simulink model "can_simple_block_bu11142"  (R2016b)
settings: Solver=FixedStepDiscrete  StartTime=0.0  StopTime=1000  FixedStep=0.2  RelTol=1e-3  EnableMultiTasking=on
undefined symbols (not defined in the file or in its folder): A, A10, A14, B, B11, B12, B13, B8, C, CS0, D, D11, D4, F3, F4, G3, G4, H3, H4, K17, K4, L3, N16, PA11, PA12, PD0, PE14, PE15, R10, R14, SCK, SIN, SOUT, T14
libraries: rappid_564xl_ec_toolbox x24
(part 1 of 2)
settings Model: Creator=RMuradov  LastModifiedBy=eugkim01
settings SolverCC: AutoInsertRateTranBlk=on
settings DataIOCC: ExternalInput=off  InitialState=off  LimitDataPoints=on  SaveFormat=Array  SignalLoggingSaveFormat=ModelDataLogs  SaveOutput=off  SignalLogging=off  SaveTime=off
settings OptimizationCC: DefaultParameterBehavior=Inlined  UseDivisionForNetSlopeComputation=on  UseFloatMulNetSlope=on  UseSpecifiedMinMax=on  InlineInvariantSignals=on  PassReuseOutputArgsAs=Individual arguments  ExpressionDepthLimit=2147483647  ZeroExternalMemoryAtStartup=off  ZeroInternalMemoryAtStartup=off  NoFixptDivByZeroProtection=on  EfficientFloat2IntCast=on  LifeSpan=1
settings DebuggingCC: UnderspecifiedInitializationDetection=Classic  MergeDetectMultiDrivingBlocksExec=none  SolverPrmCheckMsg=warning  InheritedTsInSrcMsg=none  SingleTaskRateTransMsg=error  ParameterTunabilityLossMsg=error  FcnCallInpInsideContextMsg=warning  UnconnectedInputMsg=error  UnconnectedOutputMsg=error  UnconnectedLineMsg=error  UnknownTsInhSupMsg=error  StateNameClashWarn=warning  SFUnexpectedBacktrackingDiag=warning  SFNoUnconditionalDefaultTransitionDiag=warning  SFExecutionAtInitializationDiag=none
settings HardwareCC: ProdBitPerPointer=32  ProdBitPerSizeT=32  ProdBitPerPtrDiffT=32  ProdLargestAtomicInteger=Long  ProdLargestAtomicFloat=Double  ProdEndianess=BigEndian  ProdWordSize=32  ProdHWDeviceType=Freescale->32-bit PowerPC
settings ModelReferenceCC: PropagateSignalLabelsOutOfModel=off
settings RTWCC: SystemTargetFile=rappid564xl.tlc  MakeCommand=rappid_564xl_make_rtw  TemplateMakefile=rappid_564xl_default_tmf  PostCodeGenCommand=rappid_analyzegencode(buildInfo)  Description=RAppID Toolbox MPC564xL Code Generation Target (rappid)  GenerateReport=on  TLCAssert=on  BuildConfiguration=Faster Runs  IncludeHyperlinkInReport=on  LaunchReport=on  GenerateTraceInfo=on  GenerateTraceReport=on  GenerateTraceReportSl=on  GenerateTraceReportSf=on  GenerateTraceReportEml=on  GenerateCodeMetricsReport=on
settings CodeAppCC: ForceParamTrailComments=on  IgnoreCustomStorageClasses=off  OperatorAnnotations=on  SimulinkDataObjDesc=on  SFDataObjDesc=on  MATLABFcnDesc=on  CustomSymbolStrGlobalVar=rt$N$M  CustomSymbolStrType=$N$M  CustomSymbolStrFcn=$N$M$F  CustomSymbolStrMacro=$N$M  InsertBlockDesc=on  MATLABSourceComments=on  InternalIdentifier=Classic
settings STFCustomTargetCC: CombineOutputUpdateFcns=on  CombineSignalStateStructs=on  ERTCustomFileBanners=on  SupportAbsoluteTime=off  SupportComplex=off  SupportContinuousTime=off  RemoveResetFunc=on  MATLABClassNameForMDSCustomization=Simulink.SoftwareTarget.ERTCustomization  GRTInterface=off  SystemTargetFile=rappid564xl.tlc
settings ERTTargetCC: ParMdlRefBuildCompliant=off  CompOptLevelCompliant=off  ConcurrentExecutionCompliant=off  CombineSignalStateStructs=on  ERTFirstTimeCompliant=off  SupportAbsoluteTime=off  SupportComplex=off  SupportNonInlinedSFcns=on  ModelStepFunctionPrototypeControlCompliant=off  CPPClassGenCompliant=off  UseToolchainInfoCompliant=off  InlinedParameterPlacement=NonHierarchical  ERTCustomFileTemplate=example_file_process.tlc  ERTFilePackagingFormat=CompactWithDataFile
settings ConfigComp: CovMetricSettings=dw  CovHtmlReporting=on  CovSaveCumulativeToWorkspaceVar=on  CovSaveSingleToWorkspaceVar=on  CovExternalEMLEnable=off

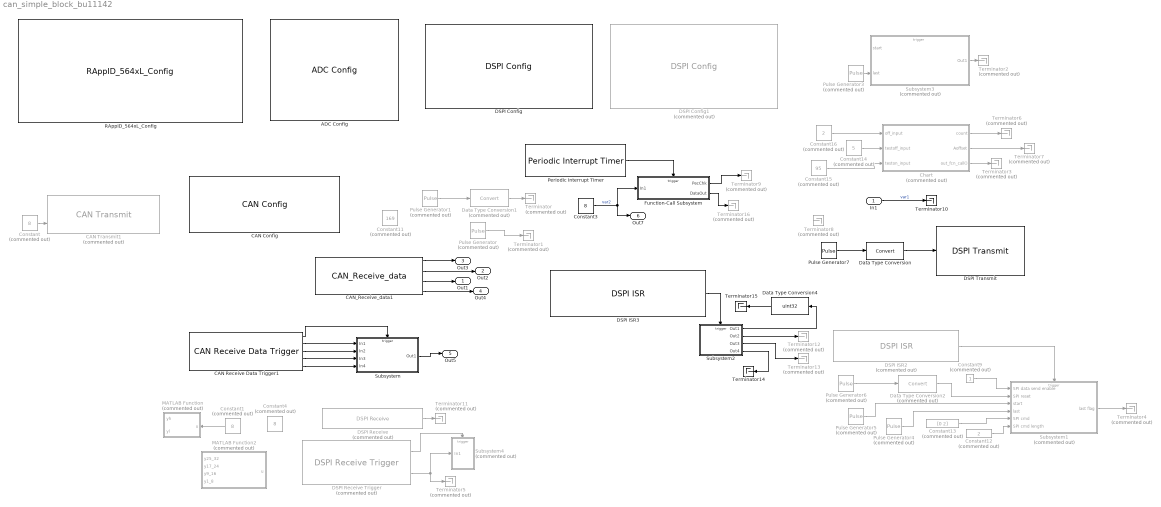
== system can_simple_block_bu11142 ==
  In1 : Inport
  ADC Config : rappid_564xl_ec_toolbox/MPC564xL/Motor Control Blocks/ADC Config  adc_unit=0  adc_ctu=off  adc_owr=on  adc_wls=Left  adc_clk=on  adc_ack=on  adc_ctr0_inp=off  adc_ctr0_shft=10 - Avin = 0  adc_ctr0_cmp=01  adc_ctr0_samp=3  adc_ctr1_inp=off  adc_ctr1_cmp=01  adc_ctr1_samp=1  adc_ctr1_tsens=PTAT  adc_pscr_preval=V0  adc_pscr_preconv=off
  CAN Config : rappid_564xl_ec_toolbox/MPC564xL/Communication Blocks/CAN Config  Priority=1  can_unit=A  can_unit_v2=0  can_idam=A - One full ID (standard or extended) per filter element.  can_srx_dis=1 - Self reception disabled  can_presdiv=4  can_rjw=3  can_pseg1=3  can_pseg2=3  can_clk_src=0 - The CAN engine clock source is the oscillator clock  can_lpb=0 - Loop Back disabled  can_smp=1 - Three samples are used to determine the value of the received bit  can_boff_rec=0 - Automatic recovering from Bus Off state enabled  can_tsyn=0 - Timer Sync feature disabled  can_lbuf=0 - Buffer with highest priority is transmitted first  can_lom=0 - Listen Only Mode is deactivated  can_propseg=6
  CAN Receive Data Trigger1 : rappid_564xl_ec_toolbox/MPC564xL/Communication Blocks/CAN Receive Data Trigger  can_unit=A  can_unit_v2=0  can_buffer=5  can_id=1021  can_isr_prio=14
  CAN Transmit1 : rappid_564xl_ec_toolbox/MPC564xL/Communication Blocks/CAN Transmit  Commented=on  can_unit=A  can_unit_v2=0  can_buffer=14  can_id=522
  CAN_Receive_data1 : rappid_564xl_ec_toolbox/MPC564xL/Communication Blocks/CAN_Receive_data  can_unit=A  can_unit_v2=0  can_buffer=7  can_id=1010
  Chart : Stateflow chart  Commented=on  TreatAsAtomicUnit=on
  Constant : Constant  Commented=on  Value=8  OutDataTypeStr=uint8
  Constant1 : Constant  Commented=on  Value=8  OutDataTypeStr=uint16
  Constant11 : Constant  Commented=on  Value=169  OutDataTypeStr=uint16
  Constant12 : Constant  Commented=on  Value=2  OutDataTypeStr=uint8
  Constant13 : Constant  Commented=on  Value=[0 2]  OutDataTypeStr=uint8
  Constant14 : Constant  Commented=on  Value=5
  Constant15 : Constant  Commented=on  Value=95
  Constant16 : Constant  Commented=on  Value=2
  Constant3 : Constant  Value=8  OutDataTypeStr=uint16
  Constant4 : Constant  Commented=on  Value=8  OutDataTypeStr=uint16
  Constant9 : Constant  Commented=on  OutDataTypeStr=boolean
  DSPI Config : rappid_564xl_ec_toolbox/MPC564xL/Communication Blocks/DSPI Config  Priority=1  dspi_Num=1  dspi_Mode=Master  dspi_MTFE=off  dspi_CONT_SCKE=off  dspi_PCSSE=off  dspi_ROOE=off  dspi_DIS_TXF=Disable  dspi_DIS_RXF_v2=Disable  dspi_SMPL_PT=DSPI samples SIN at driving SCK edge  dspi_FMSZ=8  dspi_CPOL=High  dspi_CPHA=Data is changed on the leading edge of SCK and captured on the following edge  dspi_LSBFE=MSB first  dspi_DBR=off  dspi_PCSSCK=7  dspi_PASC=1  dspi_PDT=5  dspi_PBR=3  dspi_CSSCK=256  dspi_ASC=256  dspi_DT=8  dspi_BR=128  dspi_PCSIS0=High  dspi_PCSIS1=High  dspi_PCSIS2=High  dspi_PCSIS3=High  dspi_PCSIS4=High  dspi_PCSIS5=High  dspi_PCSIS6=High  dspi_PCSIS7=High  dspi_DIS_RXF=Oops
  DSPI Config1 : rappid_564xl_ec_toolbox/MPC564xL/Communication Blocks/DSPI Config  Priority=1  Commented=on  dspi_Num=0  dspi_Mode=Master  dspi_MTFE=off  dspi_CONT_SCKE=off  dspi_PCSSE=off  dspi_ROOE=off  dspi_DIS_TXF=Disable  dspi_DIS_RXF_v2=Disable  dspi_SMPL_PT=DSPI samples SIN at driving SCK edge  dspi_FMSZ=8  dspi_CPOL=Low  dspi_CPHA=Data is changed on the leading edge of SCK and captured on the following edge  dspi_LSBFE=MSB first  dspi_DBR=off  dspi_PCSSCK=1  dspi_PASC=1  dspi_PDT=3  dspi_PBR=1  dspi_CSSCK=8  dspi_ASC=8  dspi_DT=16  dspi_BR=2  dspi_PCSIS0=High  dspi_PCSIS1=High  dspi_PCSIS2=High  dspi_PCSIS3=High  dspi_PCSIS4=High  dspi_PCSIS5=High  dspi_PCSIS6=High  dspi_PCSIS7=High  dspi_DIS_RXF=Oops
  DSPI ISR2 : rappid_564xl_ec_toolbox/MPC564xL/Communication Blocks/DSPI ISR  Commented=on  dspi_Num=1  dspi_isr_name=TCF - Transfer Complete  dspi_isrPrio=13  dspi_isr_tfuf=off  dspi_isr_rfof=on
  DSPI ISR3 : rappid_564xl_ec_toolbox/MPC564xL/Communication Blocks/DSPI ISR  dspi_Num=1  dspi_isr_name=EOQF - End of Queue  dspi_isrPrio=11  dspi_isr_tfuf=off  dspi_isr_rfof=on
  DSPI Receive : rappid_564xl_ec_toolbox/MPC564xL/Communication Blocks/DSPI Receive  Commented=on  dspi_Num=1
  DSPI Receive Trigger : rappid_564xl_ec_toolbox/MPC564xL/Communication Blocks/DSPI Receive Trigger  Commented=on  dspi_Num=1  dspi_ISRPri=13
  DSPI Transmit : rappid_564xl_ec_toolbox/MPC564xL/Communication Blocks/DSPI Transmit  Priority=2  dspi_Num=1  dspi_CONT=off  dspi_PUSHR_PE=off  dspi_PUSHR_PP=off  dspi_PCS_0=36 : C[4] : [11] : [H3] : CS0  dspi_PCS_1=5 : A[5] : [14] : [H4] : CS0  dspi_PCS_2=3 : A[3] : [92] : [K17] : CS0  dspi_PCS_slave_0=36 : C[4] : [11] : [H3] : CS0  dspi_PCS_slave_1=5 : A[5] : [14] : [H4] : CS0  dspi_PCS_slave_2=3 : A[3] : [92] : [K17] : CS0  dspi_SIN_0=39 : C[7] : [15] : [K4] : SIN  dspi_SIN_1=8 : A[8] : [12] : [F4]  dspi_SIN_2=2 : A[2] : [84] : [N16] : SIN  dspi_SCK_0=37 : C[5] : [13] : [G3] : SCK  dspi_SCK_1=6 : A[6] : [2] : [G4] : SCK  dspi_SCK_2=0 : A[0] : [73] : [T14] : SCK  dspi_SOUT_0=38 : C[6] : [142] : [D4] : SOUT  dspi_SOUT_1=7 : A[7] : [10] : [F3] : SOUT  dspi_SOUT_2=1 : A[1] : [74] : [R14] : SOUT  dspi_Strobe=None  dspi_eoq=off  dspi_pcsx=Assert
  Data Type Conversion : DataTypeConversion  Priority=1
  Data Type Conversion1 : DataTypeConversion  Priority=1  Commented=on
  Data Type Conversion2 : DataTypeConversion  Priority=1  Commented=on
  Data Type Conversion4 : DataTypeConversion  Priority=1  OutDataTypeStr=uint32
  Function-Call Subsystem : Subsystem  TreatAsAtomicUnit=on
      settings: RTWSystemCode=Nonreusable function
  MATLAB Function : MATLAB Function  Commented=on  TreatAsAtomicUnit=on
  MATLAB Function2 : MATLAB Function  Commented=on  TreatAsAtomicUnit=on
  Periodic Interrupt Timer : rappid_564xl_ec_toolbox/MPC564xL/General Purpose Blocks/Periodic Interrupt Timer  pit_chan=1  pit_timeout=50  int_priority=12  pit_timeout_val=5999999
  Pulse Generator : DiscretePulseGenerator  Commented=on  Amplitude=9  Period=10
  Pulse Generator1 : DiscretePulseGenerator  Commented=on  Period=5  PulseWidth=3
  Pulse Generator3 : DiscretePulseGenerator  Commented=on  Period=100  PhaseDelay=5
  Pulse Generator4 : DiscretePulseGenerator  Commented=on  Period=100  PhaseDelay=5
  Pulse Generator5 : DiscretePulseGenerator  Commented=on  Period=100
  Pulse Generator6 : DiscretePulseGenerator  Commented=on  Period=10000000  PhaseDelay=1
  Pulse Generator7 : DiscretePulseGenerator  Amplitude=0  Period=100
  RAppID_564xL_Config : rappid_564xl_ec_toolbox/MPC564xL/RAppID_564xL_Config  SystemClock=120  XTAL=40  MC_clock_60=12  MC_clock_80=16  MC_clock_120=10  SWG_clock_60=20  SWG_clock_80=13.334  SWG_clock_120=20  Compiler=CodeWarrior  MemTarget=RAM  Part=MPC5643L  Package=144 LQFP  global_int_priority=11  base_tick_priority=12  sys_task_supress=off  exception_handlers=off  stored_mdl_name=can_simple_block_bu11142  freemaster_interface=Oops  freemaster_rx_pin="LINFlex_0 Rx Pin 116 : \"PB[3]\""  freemaster_tx_pin="LINFlex_0 Tx Pin 114 : \"PB[2]\""  freemaster_interface_1=None  freemaster_enable=off  freemaster_rate=57600  freemaster_tx0_pin=18 : B[2] : 114 : A14  freemaster_rx0_pin=19 : B[3] : 116 : B13  freemaster_tx1_pin=57 : D[9] : 26 : L3  freemaster_rx1_pin=29 : B[13] : 60 : R10  freemaster_can_channel=1CH  freemater_can_speed=500K  freemaster_can_msgig=0x7AA  ccp_interface=None  ccp_enable=off  ccp_can_channel=CH1 (MB 0 - 1)  ccp_can_speed=500K  ccp_can_cro_id=256  ccp_can_dto_id=257  ccp_dev_id=RappID  ccp_dev_addr=0  ccp_odt=3  ccp_daq=3  pil_enable=off  pil_bam=on  comport=6  pil_rate=57600  bam_password_def=on  bam_password=0xFEEDFACECAFEBEEF  bam_sa_cs=on  bam_start_address=0x40005000  bam_code_size=0xa000  cons_dspi=on  cons_can=on  cons_adc=on  cons_pwm=on  cons_ctu=on  cons_swg=on  cons_eTimer=on  cons_fm=on
  Subsystem : Subsystem
      settings: RTWSystemCode=Nonreusable function
  Subsystem1 : Subsystem  Commented=on
      settings: RTWSystemCode=Nonreusable function
  Subsystem2 : Subsystem
      settings: RTWSystemCode=Nonreusable function
  Subsystem3 : Subsystem  Commented=on
  Subsystem4 : Subsystem  Commented=on
      settings: RTWSystemCode=Nonreusable function
  Terminator{,1..9,11..13,16} (14 alike) : Terminator  Commented=on
  Terminator10 : Terminator
  Terminator14 : Terminator
  Terminator15 : Terminator
  Out1 : Outport
  Out2 : Outport  Port=2
  Out3 : Outport  Port=3
  Out4 : Outport  Port=4
  Out5 : Outport  Port=5
  Out7 : Outport  Port=6
  wires:
  CAN_Receive_data1/4 -> Out4/1
  CAN_Receive_data1/3 -> Out1/1
  CAN_Receive_data1/2 -> Out2/1
  CAN_Receive_data1/1 -> Out3/1
  Constant/1 -> CAN Transmit1/2
  CAN Receive Data Trigger1/3 -> Subsystem/2(In2)
  CAN Receive Data Trigger1/4 -> Subsystem/3(In3)
  CAN Receive Data Trigger1/5 -> Subsystem/4(In4)
  CAN Receive Data Trigger1/2 -> Subsystem/1(In1)
  CAN Receive Data Trigger1/1 -> Subsystem/Trigger
  Subsystem/1(Out1) -> Out5/1
  Pulse Generator1/1 -> Data Type Conversion1/1
  Data Type Conversion1/1 -> Terminator/1
  DSPI ISR2/1 -> Subsystem1/Trigger
  DSPI ISR3/1 -> Subsystem2/Trigger
  Constant9/1 -> Subsystem1/1(SPI data send enable)
  Pulse Generator/1 -> Terminator1/1
  Subsystem1/1(last flag) -> Terminator4/1
  Pulse Generator3/1 -> Subsystem3/2(last)
  Subsystem3/1(Out1) -> Terminator2/1
  Pulse Generator4/1 -> Subsystem1/4(last)
  Constant12/1 -> Subsystem1/6(SPI cmd length)
  Constant13/1 -> Subsystem1/5(SPI cmd)
  Chart/1(count) -> Terminator6/1
  Chart/2(" Aoffset") -> Terminator7/1
  Constant16/1 -> Chart/1(off_input)
  Constant14/1 -> Chart/2(testoff_input)
  Constant15/1 -> Chart/3(teston_input)
  Pulse Generator5/1 -> Subsystem1/3(start)
  Pulse Generator6/1 -> Data Type Conversion2/1
  Data Type Conversion2/1 -> Subsystem1/2(SPI reset)
  Chart/3(out_fcn_call()) -> Terminator3/1
  Periodic Interrupt Timer/1 -> Function-Call Subsystem/Trigger
  In1/1 -> Terminator10/1  "var1"
  Constant3/1 -> Function-Call Subsystem/1(In1), Out7/1  "var2"
  Data Type Conversion/1 -> DSPI Transmit/1
  Pulse Generator7/1 -> Data Type Conversion/1
  Data Type Conversion4/1 -> Terminator15/1
  DSPI Receive Trigger/2 -> Terminator5/1, Subsystem4/1(In1)
  DSPI Receive Trigger/1 -> Subsystem4/Trigger
  Subsystem2/1(Out1) -> Data Type Conversion4/1
  DSPI Receive/1 -> Terminator11/1
  Subsystem2/4(Out4) -> Terminator14/1
  Subsystem2/2(Out2) -> Terminator12/1
  Subsystem2/3(Out3) -> Terminator13/1
  Constant1/1 -> MATLAB Function/1(u)
  Function-Call Subsystem/1(PecChk) -> Terminator9/1
  Function-Call Subsystem/2(DataOut) -> Terminator16/1

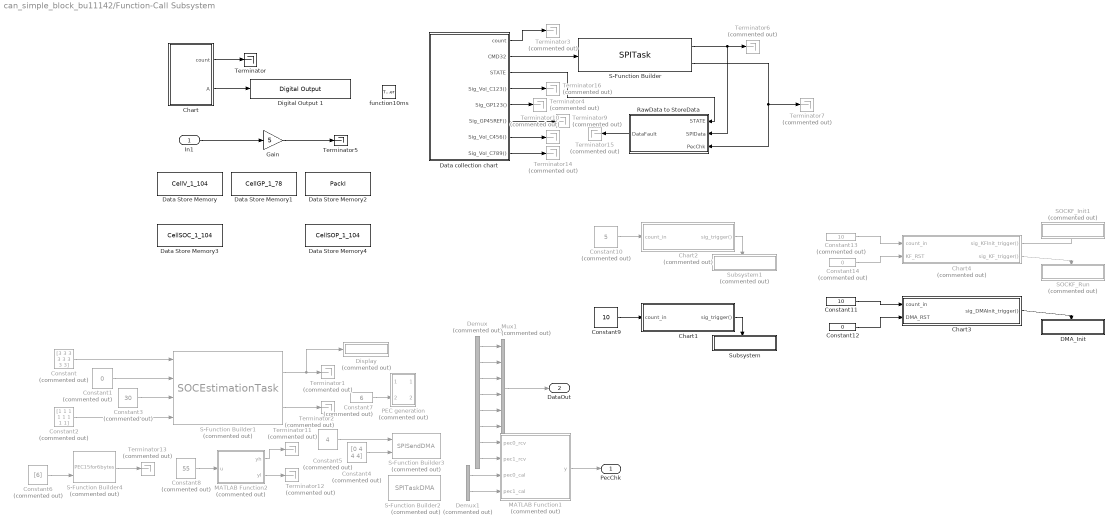
== system can_simple_block_bu11142/Function-Call Subsystem ==
  In1 : Inport
  function10ms : TriggerPort  TriggerType=function-call  VariantControl=Variant
  Chart : Stateflow chart  TreatAsAtomicUnit=on
  Chart1 : Stateflow chart  TreatAsAtomicUnit=on
  Chart2 : Stateflow chart  Commented=on  TreatAsAtomicUnit=on
  Chart3 : Stateflow chart  TreatAsAtomicUnit=on
  Chart4 : Stateflow chart  Commented=on  TreatAsAtomicUnit=on
  Constant : Constant  Commented=on  Value=[3 3 3 3 3 3 3 3]
  Constant1 : Constant  Commented=on  Value=0
  Constant10 : Constant  Commented=on  Value=5  OutDataTypeStr=Inherit: Inherit via back propagation
  Constant11 : Constant  Value=10  OutDataTypeStr=Inherit: Inherit via back propagation
  Constant12 : Constant  Value=0  OutDataTypeStr=Inherit: Inherit via back propagation
  Constant13 : Constant  Commented=on  Value=10  OutDataTypeStr=Inherit: Inherit via back propagation
  Constant14 : Constant  Commented=on  Value=0  OutDataTypeStr=Inherit: Inherit via back propagation
  Constant2 : Constant  Commented=on  Value=[1 1 1 1 1 1 1 1]  OutDataTypeStr=boolean
  Constant3 : Constant  Commented=on  Value=30
  Constant4 : Constant  Commented=on  Value=[0 4 4 4]  OutDataTypeStr=Inherit: Inherit via back propagation
  Constant5 : Constant  Commented=on  Value=4  OutDataTypeStr=Inherit: Inherit via back propagation
  Constant6 : Constant  Commented=on  Value=[6]  OutDataTypeStr=Inherit: Inherit via back propagation
  Constant7 : Constant  Commented=on  Value=6  OutDataTypeStr=Inherit: Inherit via back propagation
  Constant8 : Constant  Commented=on  Value=55  OutDataTypeStr=Inherit: Inherit via back propagation
  Constant9 : Constant  Value=10  OutDataTypeStr=Inherit: Inherit via back propagation
  DMA_Init : Subsystem
  Data Store Memory : DataStoreMemory  DataStoreName=CellV_1_104  ReadBeforeWriteMsg=warning  WriteAfterWriteMsg=warning  WriteAfterReadMsg=warning  ShowAdditionalParam=off  OutDataTypeStr=uint16  Dimensions=104
  Data Store Memory1 : DataStoreMemory  DataStoreName=CellGP_1_78  ReadBeforeWriteMsg=warning  WriteAfterWriteMsg=warning  WriteAfterReadMsg=warning  ShowAdditionalParam=off  OutDataTypeStr=int16  Dimensions=78
  Data Store Memory2 : DataStoreMemory  DataStoreName=PackI  ReadBeforeWriteMsg=warning  WriteAfterWriteMsg=warning  WriteAfterReadMsg=warning  ShowAdditionalParam=off  OutDataTypeStr=int32  Dimensions=1
  Data Store Memory3 : DataStoreMemory  DataStoreName=CellSOC_1_104  ReadBeforeWriteMsg=warning  WriteAfterWriteMsg=warning  WriteAfterReadMsg=warning  ShowAdditionalParam=off  OutDataTypeStr=uint16  Dimensions=104
  Data Store Memory4 : DataStoreMemory  DataStoreName=CellSOP_1_104  ReadBeforeWriteMsg=warning  WriteAfterWriteMsg=warning  WriteAfterReadMsg=warning  ShowAdditionalParam=off  OutDataTypeStr=int16  Dimensions=104
  Data collection chart : Stateflow chart  TreatAsAtomicUnit=on
  Demux : Demux  Commented=on  Outputs=8
  Demux1 : Demux  Commented=on  Outputs=2
  Digital Output 1 : rappid_564xl_ec_toolbox/MPC564xL/General Purpose Blocks/Digital Output   gpio_outputs="78  : PE14 : [ 119 ] : [ B12 ]"  pinNum=[ 119 ]  pcrNum=78
  Display : Display  Commented=on
  Gain : Gain  Gain=5
  MATLAB Function1 : MATLAB Function  Commented=on  TreatAsAtomicUnit=on
  MATLAB Function2 : MATLAB Function  Commented=on  TreatAsAtomicUnit=on
  Mux1 : Mux  Commented=on  Inputs=6
  PEC generation : MATLAB Function  Commented=on  TreatAsAtomicUnit=on
  RawData to StoreData : MATLAB Function  TreatAsAtomicUnit=on
  S-Function Builder : S-Function  InitFcn=try, set_param(gcb,'FunctionName','SPITask'), end  FunctionName=SPITask  SFunctionModules=SPITask_wrapper BMU_Driver  SFunctionDeploymentMode=off  EnableBusSupport=off  mask(S-Function Builder){}
      mask help: Simulink:masks:SFunctionBuilder_MD
      mask init:
      | val = [[.9  0.75 0.75 1 1 .9 .9 1]',[1 1 0.75 0.75 .9 .9 1 .9]'];try , sys = get_param(gcb,'SfunBuilderFcnName');if isempty(sys), sys = get_param(gcb,'FunctionName'); end,catch, sys = get_param(gcb,'FunctionName'); end
      settings: CopyFcn=set_param(gcbh,'LinkStatus','none')  PreSaveFcn=try, set_param(gcb,'FunctionName','SPITask'), end  OpenFcn=sfunctionwizard(gcbh)
      mask Display: plot(val(:,1),val(:,2)),disp(sys), port_label('input',1,'CMD32'), port_label('output',1,'y0'), port_label('output',2,'PecChk')
  S-Function Builder1 : S-Function  Commented=on  InitFcn=try, set_param(gcb,'FunctionName','SOCEstimationTask'), end  FunctionName=SOCEstimationTask  SFunctionModules=SOCEstimationTask_wrapper Extended look2_binlx rtGetNaN rtGetInf rt_nonfinite const_params  SFunctionDeploymentMode=off  EnableBusSupport=off  mask(S-Function Builder){}
      mask help: Simulink:masks:SFunctionBuilder_MD
      mask init: same as can_simple_block_bu11142/Function-Call Subsystem/S-Function Builder
      settings: CopyFcn=set_param(gcbh,'LinkStatus','none')  PreSaveFcn=try, set_param(gcb,'FunctionName','SOCEstimationTask'), end  OpenFcn=sfunctionwizard(gcbh)
      mask Display: plot(val(:,1),val(:,2)),disp(sys), port_label('input',1,'I'), port_label('input',2,'V8'), port_label('input',3,'T'), port_label('input',4,'Enable8'), port_label('output',1,'SOC'), port_label('output',2,'Vt')
  S-Function Builder2 : S-Function  Commented=on  InitFcn=try, set_param(gcb,'FunctionName','SPITaskDMA'), end  FunctionName=SPITaskDMA  SFunctionModules=SPITaskDMA_wrapper BMU_Driver  SFunctionDeploymentMode=off  EnableBusSupport=off  mask(S-Function Builder){}
      mask help: Simulink:masks:SFunctionBuilder_MD
      mask init: same as can_simple_block_bu11142/Function-Call Subsystem/S-Function Builder
      settings: CopyFcn=set_param(gcbh,'LinkStatus','none')  PreSaveFcn=try, set_param(gcb,'FunctionName','SPITaskDMA'), end  OpenFcn=sfunctionwizard(gcbh)
      mask Display: plot(val(:,1),val(:,2)),disp(sys), port_label('output',1,'y0')
  S-Function Builder3 : S-Function  Commented=on  InitFcn=try, set_param(gcb,'FunctionName','SPISendDMA'), end  FunctionName=SPISendDMA  SFunctionModules=SPISendDMA_wrapper DMA  SFunctionDeploymentMode=off  EnableBusSupport=off  mask(S-Function Builder){}
      mask help: Simulink:masks:SFunctionBuilder_MD
      mask init: same as can_simple_block_bu11142/Function-Call Subsystem/S-Function Builder
      settings: CopyFcn=set_param(gcbh,'LinkStatus','none')  PreSaveFcn=try, set_param(gcb,'FunctionName','SPISendDMA'), end  OpenFcn=sfunctionwizard(gcbh)
      mask Display: plot(val(:,1),val(:,2)),disp(sys), port_label('input',1,'len'), port_label('input',2,'data')
  S-Function Builder4 : S-Function  Commented=on  InitFcn=try, set_param(gcb,'FunctionName','PEC15for6bytes'), end  FunctionName=PEC15for6bytes  SFunctionModules=PEC15for6bytes_wrapper BMU_Driver  SFunctionDeploymentMode=off  EnableBusSupport=off  mask(S-Function Builder){}
      mask help: Simulink:masks:SFunctionBuilder_MD
      mask init: same as can_simple_block_bu11142/Function-Call Subsystem/S-Function Builder
      settings: CopyFcn=set_param(gcbh,'LinkStatus','none')  PreSaveFcn=try, set_param(gcb,'FunctionName','PEC15for6bytes'), end  OpenFcn=sfunctionwizard(gcbh)
      mask Display: plot(val(:,1),val(:,2)),disp(sys), port_label('input',1,'data'), port_label('input',2,'len'), port_label('output',1,'y0')
  SOCKF_Init1 : Subsystem  Commented=on
  SOCKF_Run : Subsystem  Commented=on
  Subsystem : Subsystem
  Subsystem1 : Subsystem  Commented=on
  Terminator : Terminator
  Terminator{1..4,6..7,9..16} (14 alike) : Terminator  Commented=on
  Terminator5 : Terminator
  PecChk : Outport
  DataOut : Outport  Port=2
  wires:
  In1/1 -> Gain/1
  Gain/1 -> Terminator5/1
  Chart/2(" A") -> Digital Output 1/1
  Chart/1(count) -> Terminator/1
  S-Function Builder/1 -> RawData to StoreData/2(SPIData), Terminator6/1
  S-Function Builder1/1 -> Terminator1/1, Display/1
  S-Function Builder1/2 -> Terminator2/1
  Constant/1 -> S-Function Builder1/1
  Constant1/1 -> S-Function Builder1/2
  Constant2/1 -> S-Function Builder1/4
  Constant3/1 -> S-Function Builder1/3
  Constant4/1 -> S-Function Builder3/2
  Constant5/1 -> S-Function Builder3/1
  Constant6/1 -> S-Function Builder4/2
  Demux/7 -> MATLAB Function1/1(pec0_rcv)
  Demux/8 -> MATLAB Function1/2(pec1_rcv)
  MATLAB Function1/1(y) -> PecChk/1
  Demux/1 -> Mux1/1
  Demux/2 -> Mux1/2
  Demux/3 -> Mux1/3
  Demux/4 -> Mux1/4
  Demux/5 -> Mux1/5
  Demux/6 -> Mux1/6
  S-Function Builder4/1 -> Terminator13/1
  Mux1/1 -> DataOut/1
  Constant7/1 -> PEC generation/2(len)
  MATLAB Function2/1(yh) -> Terminator11/1
  MATLAB Function2/2(yl) -> Terminator12/1
  Constant8/1 -> MATLAB Function2/1(u)
  S-Function Builder/2 -> Terminator7/1, RawData to StoreData/3(PecChk)
  Demux1/1 -> MATLAB Function1/3(pec0_cal)
  Demux1/2 -> MATLAB Function1/4(pec1_cal)
  Data collection chart/1(count) -> Terminator3/1
  Data collection chart/2(CMD32) -> S-Function Builder/1
  Data collection chart/3(STATE) -> RawData to StoreData/1(STATE)
  Data collection chart/5(Sig_GP123()) -> Terminator4/1
  Data collection chart/6(Sig_GP45REF()) -> Terminator9/1
  Data collection chart/7(Sig_Vol_C456()) -> Terminator10/1
  Data collection chart/8(Sig_Vol_C789()) -> Terminator14/1
  RawData to StoreData/1(DataFault) -> Terminator15/1
  Data collection chart/4(Sig_Vol_C123()) -> Terminator16/1
  Constant9/1 -> Chart1/1(count_in)
  Chart1/1(sig_trigger()) -> Subsystem/Trigger
  Constant10/1 -> Chart2/1(count_in)
  Chart2/1(sig_trigger()) -> Subsystem1/Trigger
  Chart3/1(sig_DMAInit_trigger()) -> DMA_Init/Trigger
  Constant11/1 -> Chart3/1(count_in)
  Constant12/1 -> Chart3/2(DMA_RST)
  Chart4/1(sig_KFInit_trigger()) -> SOCKF_Init1/Trigger
  Constant13/1 -> Chart4/1(count_in)
  Constant14/1 -> Chart4/2(KF_RST)
  Chart4/2(sig_KF_trigger()) -> SOCKF_Run/Trigger

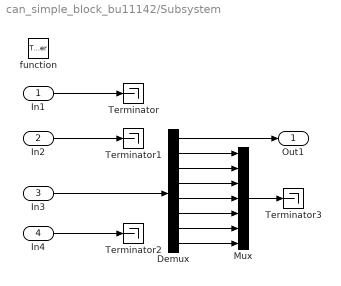
== system can_simple_block_bu11142/Subsystem ==
  In1 : Inport
  In2 : Inport  Port=2
  In3 : Inport  Port=3
  In4 : Inport  Port=4
  function : TriggerPort  TriggerType=function-call  VariantControl=Variant
  Demux : Demux  Outputs=8
  Mux : Mux  Inputs=7
  Terminator{,1..3} (4 alike) : Terminator
  Out1 : Outport
  wires:
  In1/1 -> Terminator/1
  In2/1 -> Terminator1/1
  In4/1 -> Terminator2/1
  In3/1 -> Demux/1
  Demux/8 -> Mux/7
  Demux/7 -> Mux/6
  Demux/6 -> Mux/5
  Demux/5 -> Mux/4
  Demux/4 -> Mux/3
  Demux/3 -> Mux/2
  Demux/2 -> Mux/1
  Mux/1 -> Terminator3/1
  Demux/1 -> Out1/1

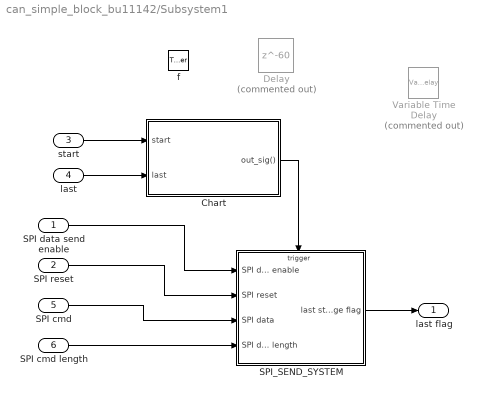
== system can_simple_block_bu11142/Subsystem1 ==
  SPI data send enable : Inport
  SPI reset : Inport  Port=2
  start : Inport  Port=3
  last : Inport  Port=4
  SPI cmd : Inport  Port=5
  SPI cmd length : Inport  Port=6
  f : TriggerPort  TriggerType=function-call  VariantControl=Variant
  Chart : Stateflow chart  TreatAsAtomicUnit=on
  Delay : Delay  Commented=on  DelayLength=60  InitialCondition=0
  SPI_SEND_SYSTEM : Subsystem
  Variable Time Delay : VariableTransportDelay  Commented=on  MaximumDelay=10
  last flag : Outport
  wires:
  SPI data send enable/1 -> SPI_SEND_SYSTEM/1(SPI data send enable)
  SPI reset/1 -> SPI_SEND_SYSTEM/2(SPI reset)
  SPI_SEND_SYSTEM/1(last stage flag) -> last flag/1
  start/1 -> Chart/1(start)
  last/1 -> Chart/2(last)
  SPI cmd/1 -> SPI_SEND_SYSTEM/3(SPI data)
  SPI cmd length/1 -> SPI_SEND_SYSTEM/4(SPI data length)
  Chart/1(out_sig()) -> SPI_SEND_SYSTEM/Trigger

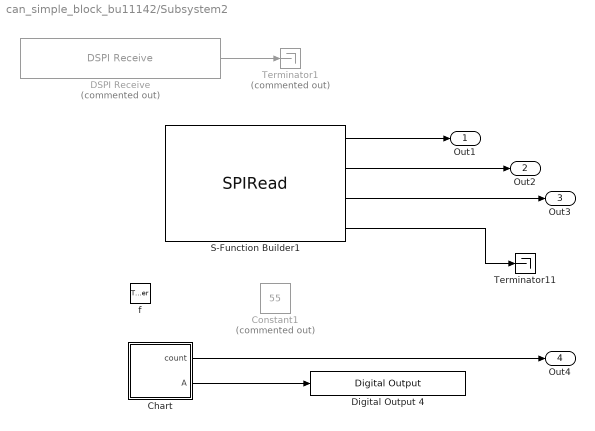
== system can_simple_block_bu11142/Subsystem2 ==
  f : TriggerPort  TriggerType=function-call  VariantControl=Variant
  Chart : Stateflow chart  TreatAsAtomicUnit=on
  Constant1 : Constant  Commented=on  Value=55  OutDataTypeStr=uint16
  DSPI Receive : rappid_564xl_ec_toolbox/MPC564xL/Communication Blocks/DSPI Receive  Commented=on  dspi_Num=1
  Digital Output 4 : rappid_564xl_ec_toolbox/MPC564xL/General Purpose Blocks/Digital Output   gpio_outputs="12  : PA12 : [ 122 ] : [ A10 ]"  pinNum=[ 122 ]  pcrNum=12
  S-Function Builder1 : S-Function  InitFcn=try, set_param(gcb,'FunctionName','SPIRead'), end  FunctionName=SPIRead  SFunctionModules=SPIRead_wrapper BMU_Driver  SFunctionDeploymentMode=off  EnableBusSupport=off  mask(S-Function Builder){}
      mask help: Simulink:masks:SFunctionBuilder_MD
      mask init: same as can_simple_block_bu11142/Function-Call Subsystem/S-Function Builder
      settings: CopyFcn=set_param(gcbh,'LinkStatus','none')  PreSaveFcn=try, set_param(gcb,'FunctionName','SPIRead'), end  OpenFcn=sfunctionwizard(gcbh)
      mask Display: plot(val(:,1),val(:,2)),disp(sys), port_label('output',1,'Vc1'), port_label('output',2,'Vc2'), port_label('output',3,'Vc3'), port_label('output',4,'PEC')
  Terminator1 : Terminator  Commented=on
  Terminator11 : Terminator
  Out1 : Outport
  Out2 : Outport  Port=2
  Out3 : Outport  Port=3
  Out4 : Outport  Port=4
  wires:
  Chart/2(" A") -> Digital Output 4/1
  Chart/1(count) -> Out4/1
  DSPI Receive/1 -> Terminator1/1
  S-Function Builder1/1 -> Out1/1
  S-Function Builder1/2 -> Out2/1
  S-Function Builder1/3 -> Out3/1
  S-Function Builder1/4 -> Terminator11/1

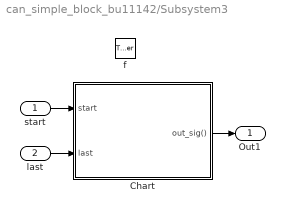
== system can_simple_block_bu11142/Subsystem3 ==
  start : Inport
  last : Inport  Port=2
  f : TriggerPort  TriggerType=function-call  VariantControl=Variant
  Chart : Stateflow chart  TreatAsAtomicUnit=on
  Out1 : Outport
  wires:
  start/1 -> Chart/1(start)
  last/1 -> Chart/2(last)
  Chart/1(out_sig()) -> Out1/1

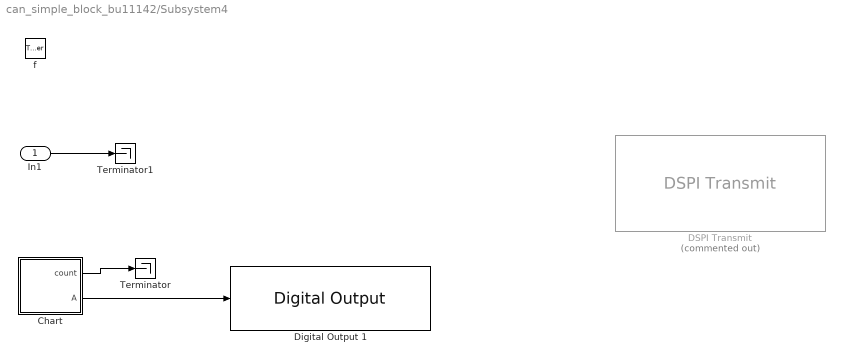
== system can_simple_block_bu11142/Subsystem4 ==
  In1 : Inport
  f : TriggerPort  TriggerType=function-call  VariantControl=Variant
  Chart : Stateflow chart  TreatAsAtomicUnit=on
  DSPI Transmit : rappid_564xl_ec_toolbox/MPC564xL/Communication Blocks/DSPI Transmit  Priority=2  Commented=on  dspi_Num=0  dspi_CONT=off  dspi_PUSHR_PE=off  dspi_PUSHR_PP=off  dspi_PCS_0=36 : C[4] : [11] : [H3] : CS0  dspi_PCS_1=5 : A[5] : [14] : [H4] : CS0  dspi_PCS_2=3 : A[3] : [92] : [K17] : CS0  dspi_PCS_slave_0=36 : C[4] : [11] : [H3] : CS0  dspi_PCS_slave_1=5 : A[5] : [14] : [H4] : CS0  dspi_PCS_slave_2=3 : A[3] : [92] : [K17] : CS0  dspi_SIN_0=39 : C[7] : [15] : [K4] : SIN  dspi_SIN_1=8 : A[8] : [12] : [F4]  dspi_SIN_2=2 : A[2] : [84] : [N16] : SIN  dspi_SCK_0=37 : C[5] : [13] : [G3] : SCK  dspi_SCK_1=6 : A[6] : [2] : [G4] : SCK  dspi_SCK_2=0 : A[0] : [73] : [T14] : SCK  dspi_SOUT_0=38 : C[6] : [142] : [D4] : SOUT  dspi_SOUT_1=7 : A[7] : [10] : [F3] : SOUT  dspi_SOUT_2=1 : A[1] : [74] : [R14] : SOUT  dspi_Strobe=None  dspi_eoq=off  dspi_pcsx=Assert
  Digital Output 1 : rappid_564xl_ec_toolbox/MPC564xL/General Purpose Blocks/Digital Output   gpio_outputs="79  : PE15 : [ 121 ] : [ B11 ]"  pinNum=[ 121 ]  pcrNum=79
  Terminator : Terminator
  Terminator1 : Terminator
  wires:
  In1/1 -> Terminator1/1
  Chart/1(count) -> Terminator/1
  Chart/2(" A") -> Digital Output 1/1

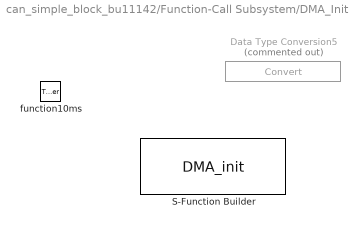
== system can_simple_block_bu11142/Function-Call Subsystem/DMA_Init ==
  function10ms : TriggerPort  TriggerType=function-call  VariantControl=Variant
  Data Type Conversion5 : DataTypeConversion  Priority=1  Commented=on
  S-Function Builder : S-Function  InitFcn=try, set_param(gcb,'FunctionName','DMA_init'), end  FunctionName=DMA_init  SFunctionModules=DMA_init_wrapper DMA  SFunctionDeploymentMode=off  EnableBusSupport=off  mask(S-Function Builder){}
      mask help: Simulink:masks:SFunctionBuilder_MD
      mask init: same as can_simple_block_bu11142/Function-Call Subsystem/S-Function Builder
      settings: CopyFcn=set_param(gcbh,'LinkStatus','none')  PreSaveFcn=try, set_param(gcb,'FunctionName','DMA_init'), end  OpenFcn=sfunctionwizard(gcbh)
      mask Display:
      | plot(val(:,1),val(:,2))
      | disp(sys)

== system can_simple_block_bu11142/Function-Call Subsystem/SOCKF_Init1 ==
  function10ms : TriggerPort  TriggerType=function-call  VariantControl=Variant
  Data Type Conversion5 : DataTypeConversion  Priority=1  Commented=on
  S-Function Builder1 : S-Function  InitFcn=try, set_param(gcb,'FunctionName','SOCEstimationInit'), end  FunctionName=SOCEstimationInit  SFunctionModules=SOCEstimationInit_wrapper Extended look2_binlx rtGetNaN rtGetInf rt_nonfinite const_params rt_roundd_snf  SFunctionDeploymentMode=off  EnableBusSupport=off  mask(S-Function Builder){}
      mask help: Simulink:masks:SFunctionBuilder_MD
      mask init: same as can_simple_block_bu11142/Function-Call Subsystem/S-Function Builder
      settings: CopyFcn=set_param(gcbh,'LinkStatus','none')  PreSaveFcn=try, set_param(gcb,'FunctionName','SOCEstimationInit'), end  OpenFcn=sfunctionwizard(gcbh)
      mask Display:
      | plot(val(:,1),val(:,2))
      | disp(sys)

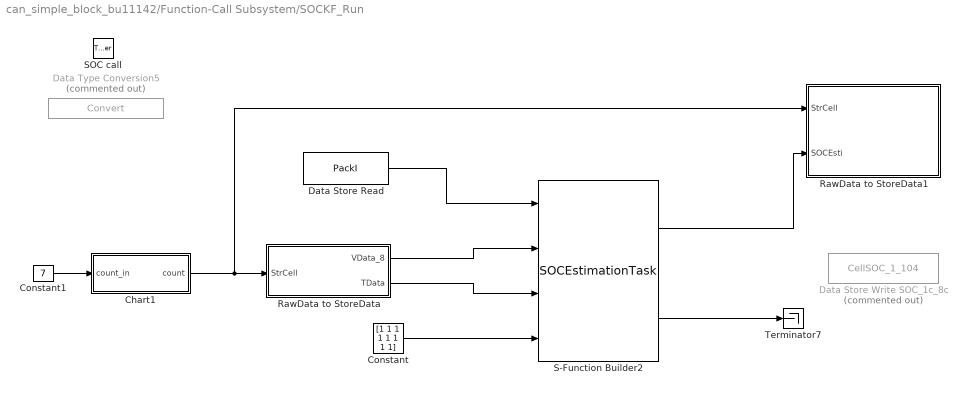
== system can_simple_block_bu11142/Function-Call Subsystem/SOCKF_Run ==
  SOC call : TriggerPort  TriggerType=function-call  VariantControl=Variant
  Chart1 : Stateflow chart  TreatAsAtomicUnit=on
  Constant : Constant  Value=[1 1 1 1 1 1 1 1]  OutDataTypeStr=Inherit: Inherit via back propagation
  Constant1 : Constant  Value=7  OutDataTypeStr=uint8
  Data Store Read : DataStoreRead  DataStoreName=PackI
  Data Store Write SOC_1c_8c : DataStoreWrite  Commented=on  DataStoreName=CellSOC_1_104
  Data Type Conversion5 : DataTypeConversion  Priority=1  Commented=on
  RawData to StoreData : MATLAB Function  TreatAsAtomicUnit=on
  RawData to StoreData1 : MATLAB Function  TreatAsAtomicUnit=on
  S-Function Builder2 : S-Function  InitFcn=try, set_param(gcb,'FunctionName','SOCEstimationTask'), end  FunctionName=SOCEstimationTask  SFunctionModules=SOCEstimationTask_wrapper Extended look2_binlx rtGetNaN rtGetInf rt_nonfinite const_params rt_roundd_snf  SFunctionDeploymentMode=off  EnableBusSupport=off  mask(S-Function Builder){}
      mask help: Simulink:masks:SFunctionBuilder_MD
      mask init: same as can_simple_block_bu11142/Function-Call Subsystem/S-Function Builder
      settings: CopyFcn=set_param(gcbh,'LinkStatus','none')  PreSaveFcn=try, set_param(gcb,'FunctionName','SOCEstimationTask'), end  OpenFcn=sfunctionwizard(gcbh)
      mask Display:
      | plot(val(:,1),val(:,2))
      | disp(sys)
      | port_label('input',1,'I')
      | port_label('input',2,'V8')
      | port_label('input',3,'T')
      | port_label('input',4,'Enable8')
      | port_label('output',1,'SOC')
      | port_label('output',2,'Vt')
  Terminator7 : Terminator
  wires:
  Constant1/1 -> Chart1/1(count_in)
  Chart1/1(count) -> RawData to StoreData1/1(StrCell), RawData to StoreData/1(StrCell)
  RawData to StoreData/1(VData_8) -> S-Function Builder2/2
  Data Store Read/1 -> S-Function Builder2/1
  RawData to StoreData/2(TData) -> S-Function Builder2/3
  Constant/1 -> S-Function Builder2/4
  S-Function Builder2/1 -> RawData to StoreData1/2(SOCEsti)
  S-Function Builder2/2 -> Terminator7/1

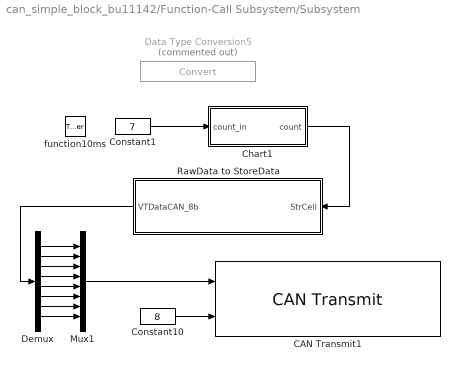
== system can_simple_block_bu11142/Function-Call Subsystem/Subsystem ==
  function10ms : TriggerPort  TriggerType=function-call  VariantControl=Variant
  CAN Transmit1 : rappid_564xl_ec_toolbox/MPC564xL/Communication Blocks/CAN Transmit  can_unit=A  can_unit_v2=0  can_buffer=14  can_id=522
  Chart1 : Stateflow chart  TreatAsAtomicUnit=on
  Constant1 : Constant  Value=7  OutDataTypeStr=uint8
  Constant10 : Constant  Value=8  OutDataTypeStr=uint8
  Data Type Conversion5 : DataTypeConversion  Priority=1  Commented=on
  Demux : Demux  Outputs=8
  Mux1 : Mux  Inputs=8
  RawData to StoreData : MATLAB Function  TreatAsAtomicUnit=on
  wires:
  Constant10/1 -> CAN Transmit1/2
  RawData to StoreData/1(VTDataCAN_8b) -> Demux/1
  Constant1/1 -> Chart1/1(count_in)
  Chart1/1(count) -> RawData to StoreData/1(StrCell)
  Demux/1 -> Mux1/1
  Demux/2 -> Mux1/2
  Demux/3 -> Mux1/3
  Demux/4 -> Mux1/4
  Demux/5 -> Mux1/5
  Demux/6 -> Mux1/6
  Demux/8 -> Mux1/8
  Demux/7 -> Mux1/7
  Mux1/1 -> CAN Transmit1/1

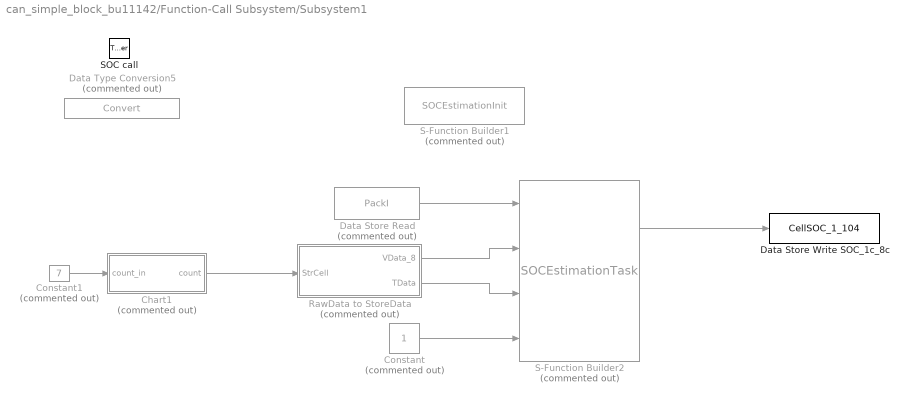
== system can_simple_block_bu11142/Function-Call Subsystem/Subsystem1 ==
  SOC call : TriggerPort  TriggerType=function-call  VariantControl=Variant
  Chart1 : Stateflow chart  Commented=on  TreatAsAtomicUnit=on
  Constant : Constant  Commented=on
  Constant1 : Constant  Commented=on  Value=7  OutDataTypeStr=uint8
  Data Store Read : DataStoreRead  Commented=on  DataStoreName=PackI
  Data Store Write SOC_1c_8c : DataStoreWrite  DataStoreName=CellSOC_1_104
  Data Type Conversion5 : DataTypeConversion  Priority=1  Commented=on
  RawData to StoreData : MATLAB Function  Commented=on  TreatAsAtomicUnit=on
  S-Function Builder1 : S-Function  Commented=on  InitFcn=try, set_param(gcb,'FunctionName','SOCEstimationInit'), end  FunctionName=SOCEstimationInit  SFunctionModules=SOCEstimationInit_wrapper Extended look2_binlx rtGetNaN rtGetInf rt_nonfinite const_params rt_roundd_snf  SFunctionDeploymentMode=off  EnableBusSupport=off  mask(S-Function Builder){}
      mask help: Simulink:masks:SFunctionBuilder_MD
      mask init: same as can_simple_block_bu11142/Function-Call Subsystem/S-Function Builder
      settings: CopyFcn=set_param(gcbh,'LinkStatus','none')  PreSaveFcn=try, set_param(gcb,'FunctionName','SOCEstimationInit'), end  OpenFcn=sfunctionwizard(gcbh)
      mask Display:
      | plot(val(:,1),val(:,2))
      | disp(sys)
  S-Function Builder2 : S-Function  Commented=on  InitFcn=try, set_param(gcb,'FunctionName','SOCEstimationTask'), end  FunctionName=SOCEstimationTask  SFunctionModules=SOCEstimationTask_wrapper Extended look2_binlx rtGetNaN rtGetInf rt_nonfinite const_params rt_roundd_snf  SFunctionDeploymentMode=off  EnableBusSupport=off  mask(S-Function Builder){}
      mask help: Simulink:masks:SFunctionBuilder_MD
      mask init: same as can_simple_block_bu11142/Function-Call Subsystem/S-Function Builder
      settings: CopyFcn=set_param(gcbh,'LinkStatus','none')  PreSaveFcn=try, set_param(gcb,'FunctionName','SOCEstimationTask'), end  OpenFcn=sfunctionwizard(gcbh)
      mask Display: plot(val(:,1),val(:,2)),disp(sys), port_label('input',1,'I'), port_label('input',2,'V8'), port_label('input',3,'T'), port_label('input',4,'Enable8'), port_label('output',1,'SOC'), port_label('output',2,'Vt')
  wires:
  Constant1/1 -> Chart1/1(count_in)
  Chart1/1(count) -> RawData to StoreData/1(StrCell)
  RawData to StoreData/1(VData_8) -> S-Function Builder2/2
  Data Store Read/1 -> S-Function Builder2/1
  RawData to StoreData/2(TData) -> S-Function Builder2/3
  Constant/1 -> S-Function Builder2/4
  S-Function Builder2/1 -> Data Store Write SOC_1c_8c/1

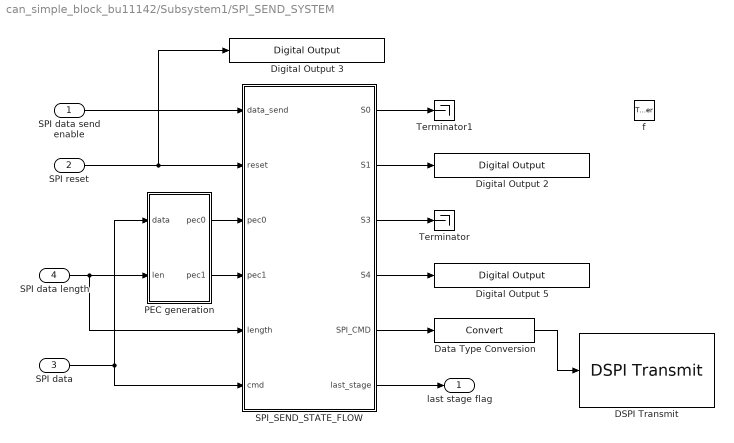
== system can_simple_block_bu11142/Subsystem1/SPI_SEND_SYSTEM ==
  SPI data send enable : Inport
  SPI reset : Inport  Port=2
  SPI data : Inport  Port=3
  SPI data length : Inport  Port=4
  f : TriggerPort  TriggerType=function-call  VariantControl=Variant
  DSPI Transmit : rappid_564xl_ec_toolbox/MPC564xL/Communication Blocks/DSPI Transmit  Priority=2  dspi_Num=1  dspi_CONT=off  dspi_PUSHR_PE=off  dspi_PUSHR_PP=off  dspi_PCS_0=36 : C[4] : [11] : [H3] : CS0  dspi_PCS_1=5 : A[5] : [14] : [H4] : CS0  dspi_PCS_2=3 : A[3] : [92] : [K17] : CS0  dspi_PCS_slave_0=36 : C[4] : [11] : [H3] : CS0  dspi_PCS_slave_1=5 : A[5] : [14] : [H4] : CS0  dspi_PCS_slave_2=3 : A[3] : [92] : [K17] : CS0  dspi_SIN_0=39 : C[7] : [15] : [K4] : SIN  dspi_SIN_1=8 : A[8] : [12] : [F4]  dspi_SIN_2=2 : A[2] : [84] : [N16] : SIN  dspi_SCK_0=37 : C[5] : [13] : [G3] : SCK  dspi_SCK_1=6 : A[6] : [2] : [G4] : SCK  dspi_SCK_2=0 : A[0] : [73] : [T14] : SCK  dspi_SOUT_0=38 : C[6] : [142] : [D4] : SOUT  dspi_SOUT_1=7 : A[7] : [10] : [F3] : SOUT  dspi_SOUT_2=1 : A[1] : [74] : [R14] : SOUT  dspi_Strobe=None  dspi_eoq=off  dspi_pcsx=Assert
  Data Type Conversion : DataTypeConversion  Priority=1
  Digital Output 2 : rappid_564xl_ec_toolbox/MPC564xL/General Purpose Blocks/Digital Output   gpio_outputs="11  : PA11 : [ 120 ] : [ D11 ]"  pinNum=[ 120 ]  pcrNum=11
  Digital Output 3 : rappid_564xl_ec_toolbox/MPC564xL/General Purpose Blocks/Digital Output   gpio_outputs="79  : PE15 : [ 121 ] : [ B11 ]"  pinNum=[ 121 ]  pcrNum=79
  Digital Output 5 : rappid_564xl_ec_toolbox/MPC564xL/General Purpose Blocks/Digital Output   gpio_outputs="48  : PD0  : [ 125 ] : [ B8 ]"  pinNum=[ 125 ]  pcrNum=48
  PEC generation : MATLAB Function  TreatAsAtomicUnit=on
  SPI_SEND_STATE_FLOW : Stateflow chart  TreatAsAtomicUnit=on
  Terminator : Terminator
  Terminator1 : Terminator
  last stage flag : Outport
  wires:
  SPI_SEND_STATE_FLOW/4(" S4") -> Digital Output 5/1
  SPI_SEND_STATE_FLOW/5(SPI_CMD) -> Data Type Conversion/1
  SPI_SEND_STATE_FLOW/1(" S0") -> Terminator1/1
  SPI_SEND_STATE_FLOW/2(" S1") -> Digital Output 2/1
  SPI data send enable/1 -> SPI_SEND_STATE_FLOW/1(data_send)
  SPI reset/1 -> Digital Output 3/1, SPI_SEND_STATE_FLOW/2(reset)
  SPI_SEND_STATE_FLOW/3(" S3") -> Terminator/1
  Data Type Conversion/1 -> DSPI Transmit/1
  SPI_SEND_STATE_FLOW/6(last_stage) -> last stage flag/1
  SPI data/1 -> SPI_SEND_STATE_FLOW/6(cmd), PEC generation/1(data)
  SPI data length/1 -> SPI_SEND_STATE_FLOW/5(length), PEC generation/2(len)
  PEC generation/1(pec0) -> SPI_SEND_STATE_FLOW/3(pec0)
  PEC generation/2(pec1) -> SPI_SEND_STATE_FLOW/4(pec1)

== stateflow chart can_simple_block_bu11142/Subsystem2/Chart ==
  state A
  state A1
  (default) -> A : {count =0;}
  A -> A1
  A1 -> A : { count = count + 1;}
  data: count output uint16; A output boolean

== stateflow chart can_simple_block_bu11142/Subsystem1/Chart ==
  state SENDING
    du:out_sig;
    du:count=count+1;
  state READY
    en:count = 1;
  (default) -> READY : {count=1;}
  READY -> SENDING : {out_sig}
  SENDING -> READY : [count > 3]
  data: start input; last input; count local
  events: out_sig output FUNCTION_CALL_EVENT

== stateflow chart can_simple_block_bu11142/Subsystem3/Chart ==
  state SENDING
    du:out_sig;
  state READY
  (default) -> READY : {count=1;}
  READY -> SENDING : [start == 1]
  SENDING -> READY : [last == 1]
  data: start input; last input; count local
  events: out_sig output FUNCTION_CALL_EVENT

== matlab function can_simple_block_bu11142/Subsystem1/SPI_SEND_SYSTEM/PEC generation ==
  data: data input; len input; pec0 output; pec1 output
function [pec0, pec1]  = PecGen(data,len)

% data_uint8 = uint8(data);
pec15Table = [0 50585 52907 2866 55503 7510 5732 54269 62471 12702 15020 65333 ...
    11464 59729 57955 10234 44439 26638 25404 42661 30040 45249 48115 ... 
    32362 22928 39945 38715	21154	33119	17606	20468	35437	23342	40631	...
    38277	20508	33761	18040	19786	35027	44841	27312	24962	42011	30694	45695	47437	31956	63161	13088	14354	64907	11894	60399	57565	9540	702	50983	52245	2444	55921	8168	5338	53571	62405	13916	15726	63735	11018	61075	58785	8248	1986	49755	51561	3312	57101	6804	4518	54335	24146	39883	37113	21856	34461	17156	18486	36271	43605	28620	25854	41319	29338	46851	48177	31144	43243	28018	26176	41945	28708	46525	48783	31510	23788	39285	37447	22494	33827	16826	19080	36625	1404	49381	52183	3662	56755	6186	4888	54913	61819	13538	16336	64073	10676	60461	59167	8838	41491	26506	27832	43297	31452	48965	46199	29166	22036	37773	39103	23846	36571	19266	16496 ... 
    34281	3972	51741	49455	1206	55115	4818	6624	56441	64387	15898	13608	61617	9036	59093	60903	10366	63805	15524	14230	61967	8690	58475	61273	10944	3386	51363	50065	1544	54773	4204	7006	57031	21674	37171	39425	24472	35941	18940	17102	34647	41133	25908	28166	43935	30818	48635	46793	29520	20950	37967	40829	23268	35097	19584	18354	33323	42449	24648	27514	44771	32030	47239	46005	30252	64577	14808	13034	63347	9358	57623	59941	12220	2118	52703	50925	884	53385	5392	7714	56251	2808	53089	50259	458	53815	6062	7324	55557	65279	15206	12372	62925	9776	58281	59547	11522	42863	25334	27076	44125	32672	47673	45323	29842	21352	38641	40387	22618	35751	20030	17676	32917];
onemask8 = uint16(hex2dec('00FF'));
onemask8_8sft = uint16(hex2dec('FF00'));
onemask88 = uint8(hex2dec('FF'));
onemask16 = uint16(hex2dec('FFFF'));

% data_test = zeros(1,2);
remainder = uint16(16);

for i=1:len
    ii = uint16(i);
%     data_test(1,i) = data(ii);
%     address = 2;
    address = bitand( ...
        bitxor( ...
        uint8(bitsra(remainder,7)),data(ii) ), ...
        onemask88);
    remainder = bitxor(bitshift(remainder,8,'uint16'),pec15Table(address+1));
end
pec15 = uint16(bitand(bitshift(remainder,1,'uint16'),onemask16));
pec0 = uint8(bitand(pec15,onemask8));
pec1 = uint8(bitsra(bitand(pec15,onemask8_8sft),8));

== stateflow chart can_simple_block_bu11142/Subsystem1/SPI_SEND_SYSTEM/SPI_SEND_STATE_FLOW ==
  state S0 [commented out]
    du:last_stage=0;
    en: cmd_i = 1;
  state S1
    en:	cmd_i = 0;
    SPI_CMD=cmd[cmd_i];
    du:
    cmd_i = cmd_i + 1;
    SPI_CMD=cmd[cmd_i];
  state S4
    en:SPI_CMD=pec0;
  state S3
    en:SPI_CMD=pec1;
  S0 -> S1 [commented out] : [data_send == true]
  (default) -> S1 : {count =0;}
  S1 -> S0 [commented out] : [reset == true]
  S4 -> S1 : {last_stage=true;}
  S3 -> S4 [order 1] : [reset == false]
  S3 -> S1 [order 2] : [reset == true]
  S1 -> S1 [order 2] : [reset == true]
  S1 -> S3 [order 1] : after(20,msec)[cmd_i >= length-1 && reset == false]
      | {cmd_i = 1;}
  data: S0 output boolean; data_send input boolean; reset input boolean; S1 output boolean; S3 output boolean; S4 output boolean; SPI_CMD output uint16; count local double; last_stage output boolean; pec0 input uint8; pec1 input uint8; cmd_i local uint8; length input uint8; cmd input uint8

== stateflow chart can_simple_block_bu11142/Chart ==
  state Aoffset
    en:offcnt = 1;
    du:offcnt = offcnt + 1;
  state Aon
    en:testoncnt=1;
    du:testoncnt=testoncnt+1;
    du:out_fcn_call;
  state Aoff
    en:testoffcnt=1;
    du:testoffcnt=testoffcnt+1;
  (default) -> Aoffset : {count =0;}
  Aoffset -> Aon : [offcnt >= off_input]
  Aoff -> Aon : [testoffcnt >= testoff_input]
  Aon -> Aoff : [testoncnt >= teston_input]
  data: count output double; Aoffset output boolean; testcnt local double; off_input input; testoff_input input; teston_input input; offcnt local double; testoffcnt local double; testoncnt local double
  events: out_fcn_call output FUNCTION_CALL_EVENT

== stateflow chart can_simple_block_bu11142/Function-Call Subsystem/Chart ==
  state A
  state A1
  (default) -> A : {count =0;}
  A -> A1
  A1 -> A : { count = count + 1;}
  data: count output double [0..10000]; A output boolean [0..1]

== matlab function can_simple_block_bu11142/MATLAB Function ==
  data: u input; yh output; yl output
function [yh,yl] = split16to8(u)
onemask8 = uint16(hex2dec('00FF'));
onemask8_8sft = uint16(hex2dec('FF00'));

yl = uint8(bitand(u,onemask8));
yh = uint8(bitsra(bitand(u,onemask8_8sft),8));

== stateflow chart can_simple_block_bu11142/Function-Call Subsystem/Chart2 ==
  state A
    en: count = 0;
    du: count = count + 1;
  state A1
    en: count = 0;
  (default) -> A : {count =0;}
  A -> A1 : [count > count_in]{sig_trigger}
  A1 -> A
  data: count local double [0..10000]; count_in input
  events: sig_trigger output FUNCTION_CALL_EVENT

== matlab function can_simple_block_bu11142/MATLAB Function2 ==
  data: u input; y25_32 output; y17_24 output; y9_16 output; y1_8 output
function [y25_32,y17_24, y9_16,y1_8 ] = split32to8(u)
onemask8 = uint32(hex2dec('000000FF'));
onemask8_8sft = uint32(hex2dec('0000FF00'));
onemask8_16sft = uint32(hex2dec('00FF0000'));
onemask8_24sft = uint32(hex2dec('FF000000'));

y1_8 = uint8(bitand(u,onemask8));
y9_16 = uint8(bitsra(bitand(u,onemask8_8sft),8));
y17_24 = uint8(bitsra(bitand(u,onemask8_16sft),16));
y25_32 = uint8(bitsra(bitand(u,onemask8_24sft),24));

== stateflow chart can_simple_block_bu11142/Subsystem4/Chart ==
  state A
  state A1
  (default) -> A : {count =0;}
  A -> A1
  A1 -> A : { count = count + 1;}
  data: count output double; A output boolean

== matlab function can_simple_block_bu11142/Function-Call Subsystem/PEC generation ==
  data: data input; len input; pec0 output; pec1 output
function [pec0, pec1]  = PecGen(data,len)

% data_uint8 = uint8(data);
pec15Table = [0 50585 52907 2866 55503 7510 5732 54269 62471 12702 15020 65333 ...
    11464 59729 57955 10234 44439 26638 25404 42661 30040 45249 48115 ... 
    32362 22928 39945 38715	21154	33119	17606	20468	35437	23342	40631	...
    38277	20508	33761	18040	19786	35027	44841	27312	24962	42011	30694	45695	47437	31956	63161	13088	14354	64907	11894	60399	57565	9540	702	50983	52245	2444	55921	8168	5338	53571	62405	13916	15726	63735	11018	61075	58785	8248	1986	49755	51561	3312	57101	6804	4518	54335	24146	39883	37113	21856	34461	17156	18486	36271	43605	28620	25854	41319	29338	46851	48177	31144	43243	28018	26176	41945	28708	46525	48783	31510	23788	39285	37447	22494	33827	16826	19080	36625	1404	49381	52183	3662	56755	6186	4888	54913	61819	13538	16336	64073	10676	60461	59167	8838	41491	26506	27832	43297	31452	48965	46199	29166	22036	37773	39103	23846	36571	19266	16496 ... 
    34281	3972	51741	49455	1206	55115	4818	6624	56441	64387	15898	13608	61617	9036	59093	60903	10366	63805	15524	14230	61967	8690	58475	61273	10944	3386	51363	50065	1544	54773	4204	7006	57031	21674	37171	39425	24472	35941	18940	17102	34647	41133	25908	28166	43935	30818	48635	46793	29520	20950	37967	40829	23268	35097	19584	18354	33323	42449	24648	27514	44771	32030	47239	46005	30252	64577	14808	13034	63347	9358	57623	59941	12220	2118	52703	50925	884	53385	5392	7714	56251	2808	53089	50259	458	53815	6062	7324	55557	65279	15206	12372	62925	9776	58281	59547	11522	42863	25334	27076	44125	32672	47673	45323	29842	21352	38641	40387	22618	35751	20030	17676	32917];
onemask8 = uint16(hex2dec('00FF'));
onemask8_8sft = uint16(hex2dec('FF00'));
onemask88 = uint8(hex2dec('FF'));
onemask16 = uint16(hex2dec('FFFF'));

% data_test = zeros(1,2);
remainder = uint16(16);

for i=1:len
    ii = uint16(i);
%     data_test(1,i) = data(ii);
%     address = 2;
    address = bitand( ...
        bitxor( ...
        uint8(bitsra(remainder,7)),data(ii) ), ...
        onemask88);
    remainder = bitxor(  bitshift(remainder,8,'uint16'), pec15Table(address+1)  );
end
pec15 = uint16(bitand(bitshift(remainder,1,'uint16'),onemask16));
pec0 = uint8(bitand(pec15,onemask8));
pec1 = uint8(bitsra(bitand(pec15,onemask8_8sft),8));

== matlab function can_simple_block_bu11142/Function-Call Subsystem/MATLAB Function2 ==
  data: u input; yh output; yl output
function [yh,yl] = split16to8(u)
onemask8 = uint16(hex2dec('00FF'));
onemask8_8sft = uint16(hex2dec('FF00'));

yl = uint8(bitand(u,onemask8));
yh = uint8(bitsra(bitand(u,onemask8_8sft),8));

== matlab function can_simple_block_bu11142/Function-Call Subsystem/MATLAB Function1 ==
  data: pec0_rcv input uint8; pec1_rcv input uint8; y output; pec0_cal input uint8; pec1_cal input uint8
function y = comp(pec0_rcv, pec1_rcv, pec0_cal, pec1_cal)


if pec0_rcv == pec0_cal && pec1_rcv == pec1_cal
  y = 1;
else
  y = 0;  
end
